simulink model "xaui_loop"  (Simulink 7.3)
settings: Solver=ode45  StartTime=0.0  StopTime=100  RelTol=1e-3
undefined symbols (not defined in the file): ROACH
libraries: xbsIndex_r4 x38, xps_library x10
settings Model: Creator=wjm  LastModifiedBy=wjm
settings OptimizationCC: InitFltsAndDblsToZero=on

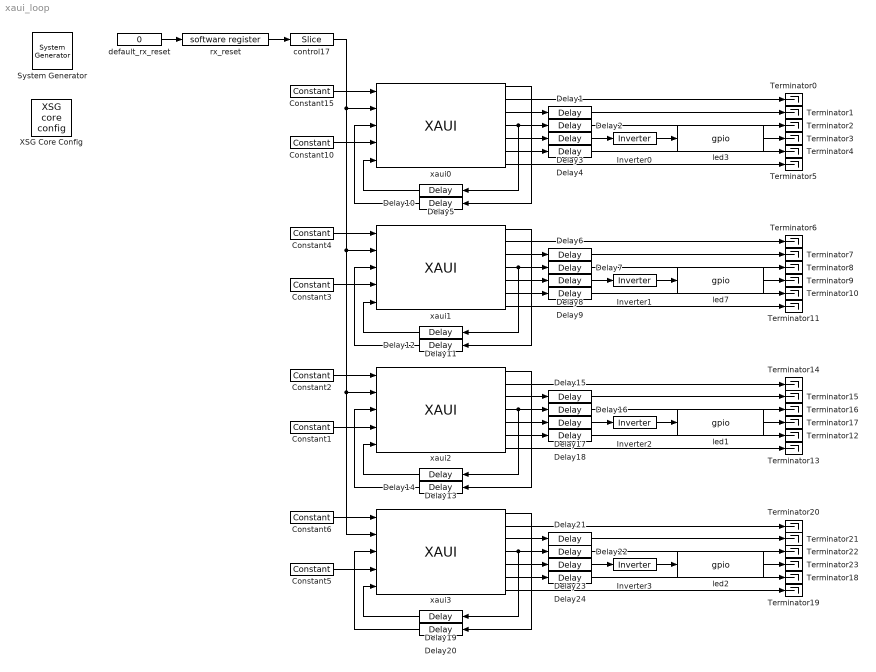
== system xaui_loop ==
  " System Generator" : xbsIndex_r4/ System Generator  Tag=genX  SystemSampleTime=-1  xilinxfamily=virtex5  part=xc5vsx95t  speed=-1  package=ff1136  synthesis_tool=XST  clock_wrapper=Clock Enables  directory=./xaui_loop/sysgen  testbench=off  simulink_period=1  sysclk_period=5  dcm_input_clock_period=100  incr_netlist=off  trim_vbits=Everywhere in SubSystem  dbl_ovrd=According to Block Masks  core_generation=According to Block Masks  run_coregen=off  deprecated_control=off  eval_field=0  block_type=sysgen
      settings: block_version=10.1.1
  Constant{1,3,5,10} (4 alike) : xbsIndex_r4/Constant  arith_type=Unsigned  const=0  n_bits=8  bin_pt=0  explicit_period=on  period=1  equ=P=C  opselect=C  inp2=PCIN>>17  opr=+  inp1=P  carry=CIN  dbl_ovrd=off  block_type=constant
      settings: block_version=10.1.1
  Constant{2,4,6,15} (4 alike) : xbsIndex_r4/Constant  arith_type=Boolean  const=1  n_bits=1  bin_pt=0  explicit_period=on  period=1  equ=P=C  opselect=C  inp2=PCIN>>17  opr=+  inp1=P  carry=CIN  dbl_ovrd=off  block_type=constant
      settings: block_version=10.1.1
  Delay{1..4,6..9,15..18,21..24} (16 alike) : xbsIndex_r4/Delay  en=off  latency=1  dbl_ovrd=off  reg_retiming=off  block_type=delay
  Delay{5,10..14,19..20} (8 alike) : xbsIndex_r4/Delay  en=off  latency=3  dbl_ovrd=off  reg_retiming=off  block_type=delay
  Inverter{0..3} (4 alike) : xbsIndex_r4/Inverter  en=off  latency=0  dbl_ovrd=off  block_type=inv
  Terminator{0..23} (24 alike) : Terminator
  XSG Core Config : xps_library/XSG core config  Tag=xps:xsg  SystemSampleTime=-1  hw_sys=ROACH:sx95t  ibob_linux=off  clk_src=sys_clk2x  iBOB_clk_src=sys_clk2x  BEE2_ctrl_clk_src=sys_clk  BEE2_usr_clk_src=sys_clk2x  ROACH_clk_src=sys_clk2x  CORR_clk_src=sys_clk  gpio_clk_io_group=iBOB:sma  gpio_clk_bit_index=0  clk_rate=200  sample_period=1  synthesis_tool=XST  mpc_type=powerpc440_ext
  control17 : xbsIndex_r4/Slice  nbits=1  boolean_output=on  mode=Lower Bit Location + Width  bit1=0  base1=MSB of Input  bit0=0  base0=LSB of Input  dbl_ovrd=off  block_type=slice
      settings: infoedit="Extracts a given range of bits from each input sample and presents it at the output.  The output type is ordinarily unsigned with binary point at zero, but can be Boolean when the slice is one bit wide.<P><P>Hardware notes: In hardware this block costs nothing."  block_version=10.1.3
  default_rx_reset : Constant  Value=0  OutDataType=sfix(16)  OutScaling=2^0  SampleTime=1
  led1 : xps_library/gpio  Tag=xps:gpio  SystemSampleTime=-1  io_group=ROACH:led  io_dir=out  arith_type=Boolean  bitwidth=1  bin_pt=0  bit_index=2  sample_period=1  use_single_ended=off  use_ddr=off  reg_iob=on  reg_clk_phase=0  termination=None
      link override convert: arith_type=Boolean  n_bits=1  bin_pt=0
  led2 : xps_library/gpio  Tag=xps:gpio  SystemSampleTime=-1  io_group=ROACH:led  io_dir=out  arith_type=Boolean  bitwidth=1  bin_pt=0  bit_index=3  sample_period=1  use_single_ended=off  use_ddr=off  reg_iob=on  reg_clk_phase=0  termination=None
      link override convert: arith_type=Boolean  n_bits=1  bin_pt=0
  led3 : xps_library/gpio  Tag=xps:gpio  SystemSampleTime=-1  io_group=ROACH:led  io_dir=out  arith_type=Boolean  bitwidth=1  bin_pt=0  bit_index=0  sample_period=1  use_single_ended=off  use_ddr=off  reg_iob=on  reg_clk_phase=0  termination=None
      link override convert: arith_type=Boolean  n_bits=1  bin_pt=0
  led7 : xps_library/gpio  Tag=xps:gpio  SystemSampleTime=-1  io_group=ROACH:led  io_dir=out  arith_type=Boolean  bitwidth=1  bin_pt=0  bit_index=1  sample_period=1  use_single_ended=off  use_ddr=off  reg_iob=on  reg_clk_phase=0  termination=None
      link override convert: arith_type=Boolean  n_bits=1  bin_pt=0
  rx_reset : xps_library/software register  Tag=xps:sw_reg  SystemSampleTime=-1  io_dir=From Processor  arith_type=Unsigned  bitwidth=32  bin_pt=0  sample_period=1  gw_name=xaui_loop_rx_reset_user_data_out
      link override xaui_loop_delay_rx_reset_user_data_out: arith_type=Unsigned  n_bits=32  bin_pt=0  period=1
      link override xaui_loop_rx_reset_user_data_out: arith_type=Unsigned  n_bits=32  bin_pt=0  period=1
  xaui0 : xps_library/XAUI  Tag=xps:xaui  SystemSampleTime=-1  demux=2  port=ROACH:0  open_phy=on  show_param=off  pre_emph=3  swing=800
      link override convert_tx_data: n_bits=32
      link override convert_tx_outofband: n_bits=4
      link override isi_correlator_xaui0_rx_data: n_bits=32
      link override isi_correlator_xaui0_rx_outofband: n_bits=4
      link override xaui_loop_delay_xaui0_rx_data: n_bits=32
      link override xaui_loop_delay_xaui0_rx_outofband: n_bits=4
      link override xaui_loop_xaui0_rx_data: n_bits=32
      link override xaui_loop_xaui0_rx_outofband: n_bits=4
  xaui1 : xps_library/XAUI  Tag=xps:xaui  SystemSampleTime=-1  demux=2  port=ROACH:1  open_phy=on  show_param=off  pre_emph=3  swing=800
      link override convert_tx_data: n_bits=32
      link override convert_tx_outofband: n_bits=4
      link override isi_correlator_xaui0_rx_data: n_bits=32
      link override isi_correlator_xaui0_rx_outofband: n_bits=4
      link override xaui_loop_delay_xaui1_rx_data: n_bits=32
      link override xaui_loop_delay_xaui1_rx_outofband: n_bits=4
      link override xaui_loop_xaui1_rx_data: n_bits=32
      link override xaui_loop_xaui1_rx_outofband: n_bits=4
  xaui2 : xps_library/XAUI  Tag=xps:xaui  SystemSampleTime=-1  demux=2  port=ROACH:2  open_phy=on  show_param=off  pre_emph=3  swing=800
      link override convert_tx_data: n_bits=32
      link override convert_tx_outofband: n_bits=4
      link override isi_correlator_xaui0_rx_data: n_bits=32
      link override isi_correlator_xaui0_rx_outofband: n_bits=4
      link override xaui_loop_delay_xaui1_rx_data: n_bits=32
      link override xaui_loop_delay_xaui1_rx_outofband: n_bits=4
      link override xaui_loop_xaui1_rx_data: n_bits=32
      link override xaui_loop_xaui1_rx_outofband: n_bits=4
      link override xaui_loop_xaui2_rx_data: n_bits=32
      link override xaui_loop_xaui2_rx_outofband: n_bits=4
  xaui3 : xps_library/XAUI  Tag=xps:xaui  SystemSampleTime=-1  demux=2  port=ROACH:3  open_phy=on  show_param=off  pre_emph=3  swing=800
      link override convert_tx_data: n_bits=32
      link override convert_tx_outofband: n_bits=4
      link override isi_correlator_xaui0_rx_data: n_bits=32
      link override isi_correlator_xaui0_rx_outofband: n_bits=4
      link override xaui_loop_delay_xaui1_rx_data: n_bits=32
      link override xaui_loop_delay_xaui1_rx_outofband: n_bits=4
      link override xaui_loop_xaui1_rx_data: n_bits=32
      link override xaui_loop_xaui1_rx_outofband: n_bits=4
      link override xaui_loop_xaui3_rx_data: n_bits=32
      link override xaui_loop_xaui3_rx_outofband: n_bits=4
  wires:
  Constant15/1 -> xaui0/1
  Constant10/1 -> xaui0/4
  xaui0/4 -> Delay2/1, Delay5/1
  xaui0/3 -> Delay1/1
  xaui0/5 -> Delay3/1
  xaui0/6 -> Delay4/1
  Delay1/1 -> Terminator1/1
  Delay3/1 -> Inverter0/1
  Constant4/1 -> xaui1/1
  Constant3/1 -> xaui1/4
  xaui1/4 -> Delay7/1, Delay11/1
  xaui1/3 -> Delay6/1
  xaui1/5 -> Delay8/1
  xaui1/6 -> Delay9/1
  Delay6/1 -> Terminator7/1
  Delay8/1 -> Inverter1/1
  default_rx_reset/1 -> rx_reset/1
  rx_reset/1 -> control17/1
  xaui1/1 -> Delay12/1
  xaui0/1 -> Delay10/1
  control17/1 -> xaui0/2, xaui1/2, xaui2/2, xaui3/2
  led3/1 -> Terminator3/1
  led7/1 -> Terminator9/1
  Delay5/1 -> xaui0/5
  Delay10/1 -> xaui0/3
  Delay11/1 -> xaui1/5
  Delay12/1 -> xaui1/3
  xaui0/2 -> Terminator0/1
  xaui0/7 -> Terminator5/1
  Delay2/1 -> Terminator2/1
  Delay4/1 -> Terminator4/1
  xaui1/2 -> Terminator6/1
  xaui1/7 -> Terminator11/1
  Delay7/1 -> Terminator8/1
  Delay9/1 -> Terminator10/1
  Inverter0/1 -> led3/1
  Inverter1/1 -> led7/1
  Constant2/1 -> xaui2/1
  Constant1/1 -> xaui2/4
  xaui2/4 -> Delay16/1, Delay13/1
  xaui2/3 -> Delay15/1
  xaui2/5 -> Delay17/1
  xaui2/6 -> Delay18/1
  Delay15/1 -> Terminator15/1
  Delay17/1 -> Inverter2/1
  xaui2/1 -> Delay14/1
  led1/1 -> Terminator17/1
  Delay13/1 -> xaui2/5
  Delay14/1 -> xaui2/3
  xaui2/2 -> Terminator14/1
  xaui2/7 -> Terminator13/1
  Delay16/1 -> Terminator16/1
  Delay18/1 -> Terminator12/1
  Inverter2/1 -> led1/1
  Constant6/1 -> xaui3/1
  Constant5/1 -> xaui3/4
  xaui3/4 -> Delay22/1, Delay19/1
  xaui3/3 -> Delay21/1
  xaui3/5 -> Delay23/1
  xaui3/6 -> Delay24/1
  Delay21/1 -> Terminator21/1
  Delay23/1 -> Inverter3/1
  xaui3/1 -> Delay20/1
  led2/1 -> Terminator23/1
  Delay19/1 -> xaui3/5
  Delay20/1 -> xaui3/3
  xaui3/2 -> Terminator20/1
  xaui3/7 -> Terminator19/1
  Delay22/1 -> Terminator22/1
  Delay24/1 -> Terminator18/1
  Inverter3/1 -> led2/1
